simulink subsystem "CurrentSensor"  (R2023a)
settings: Solver=VariableStepAuto  StartTime=0.0  StopTime=10.0  RelTol=1e-3
undefined symbols (not defined in the file): R_cur
libraries: simulink x1
settings Model: Creator=ПК  LastModifiedBy=ПК

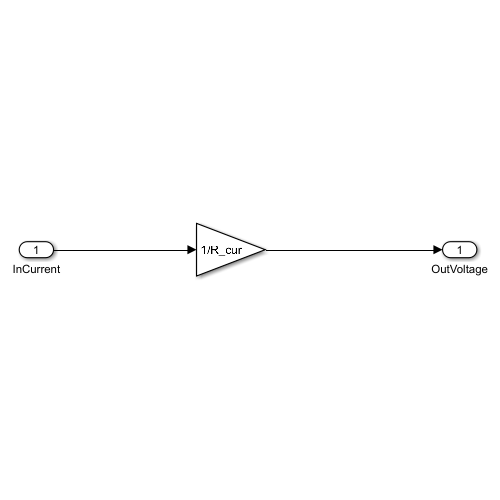
[thumbnail: Simulink's stored preview of the top-level diagram]
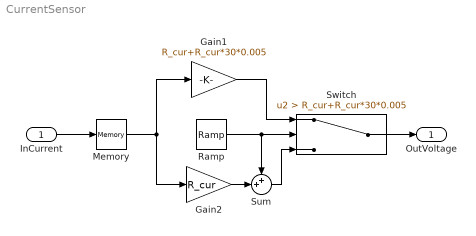
== system CurrentSensor ==
  InCurrent : Inport
  Gain1 : Gain  Gain=R_cur+R_cur*30*0.005
  Gain2 : Gain  Gain=R_cur
  Memory : Memory
  Ramp : simulink/Sources/Ramp  slope=1  start=0  InitialOutput=0
  Sum : Sum  Inputs=++|
  Switch : Switch  Criteria=u2 > Threshold  Threshold=R_cur+R_cur*30*0.005  SaturateOnIntegerOverflow=off  InputSameDT=off
  OutVoltage : Outport
  wires:
  InCurrent/1 -> Memory/1
  Switch/1 -> OutVoltage/1
  Memory/1 -> Gain1/1, Gain2/1
  Gain2/1 -> Sum/2
  Ramp/1 -> Switch/2, Sum/1
  Gain1/1 -> Switch/1
  Sum/1 -> Switch/3
